simulink model "ExampleAnimationControl"  (Simulink 9.2)
settings: Solver=FixedStepDiscrete  StartTime=0.0  StopTime=inf  FixedStep=0.001  RelTol=1e-3  EnableMultiTasking=on
libraries: rFproPhysicsLib x6
settings Model: Creator=enewton  LastModifiedBy=AkinoriMinakawa
settings Model: SuppressorTable=|
  | <?xml version="1.0" encoding="UTF-8" standalone="yes" ?>
  | <!DOCTYPE boost_serialization>
  | <boost_serialization signature="serialization::archive" version="15">
  | <DiagnosticSuppressor class_id="0" tracking_level="0" version="6">
  | 	<Table class_id="1" tracking_level="0" version="0">
  | 		<count>4</count>
  | 		<bucket_count>8</bucket_count>
  | 		<item_version>0</item_version>
  | 		<item class_id="2" tracking_level="0" version="0">
  | 			<first class_id="3" tracking_level="0" version="6">
  | 				<Source class_id="4" tracking_level="0" version="0">
  | 					<count>1</count>
  | 					<item_version>0</item_version>
  | 					<item>ExampleAnimationControl/Insert Actor - Manual (state control)/Enable Send/Subsystem/Counter Free-Running2</item>
  | 				</Source>
  | 			</first>
  | 			<second class_id="5" tracking_level="0" version="6">
  | 				<SuppressedData class_id="6" tracking_level="0" version="0">
  | 					<count>2</count>
  | 					<bucket_count>8</bucket_count>
  | 					<item_version>0</item_version>
  | 					<item class_id="7" tracking_level="0" version="0">
  | 						<first class_id="8" tracking_level="0" version="6">
  | 							<ID>SimulinkFixedPoint:util:Overflowoccurred</ID>
  | 							<Cause>
  | 								<Source>
  | 									<count>0</count>
  | 									<item_version>0</item_version>
  | 								</Source>
  | 							</Cause>
  | 						</first>
  | 						<second class_id="9" tracking_level="0" version="6">
  | 							<Comment></Comment>
  | 							<User></User>
  | 							<LastModified class_id="10" tracking_level="0" version="0">
  | 								<ptime_date class_id="11" tracking_level="0" version="0">
  | 									<date>20160523</date>
  | 								</ptime_date>
  | 								<ptime_time_duration class_id="12" tracking_level="0" version="0">
  | 									<is_special>0</is_special>
  | 									<time_duration_hours>10</time_duration_hours>
  | 									<time_duration_minutes>57</time_duration_minutes>
  | 									<time_duration_seconds>55</time_duration_seconds>
  | 									<time_duration_fractional_seconds>0</time_duration_fractional_seconds>
  | 								</ptime_time_duration>
  | 							</LastModified>
  | 							<SuppressionType>1</SuppressionType>
  | 						</second>
  | 					</item>
  | 					<item>
  | 						<first>
  | 							<ID>Simulink:DataType:WarningOverFlowDetected</ID>
  | 							<Cause>
  | 								<Source>
  | 									<count>0</count>
  | 									<item_version>0</item_version>
  | 								</Source>
  | 							</Cause>
  | 						</first>
  | 						<second>
  | 							<Comment></Comment>
  | 							<User></User>
  | 							<LastModified>
  | 								<ptime_date>
  | 									<date>20160523</date>
  | 								</ptime_date>
  | 								<ptime_time_duration>
  | 									<is_special>0</is_special>
  | 									<time_duration_hours>10</time_duration_hours>
  | 									<time_duration_minutes>57</time_duration_minutes>
  | 									<time_duration_seconds>55</time_duration_seconds>
  | 									<time_duration_fractional_seconds>0</time_duration_fractional_seconds>
  | 								</ptime_time_duration>
  | 							</LastModified>
  | 							<SuppressionType>1</SuppressionType>
  | 						</second>
  | 					</item>
  | 				</SuppressedData>
  | 			</second>
  | 		</item>
  | 		<item>
  | 			<first>
  | 				<Source>
  | 					<count>1</count>
  | 					<item_version>0</item_version>
  | 					<item>ExampleAnimationControl/Insert Actor - Hybrid/Enable Send/Subsystem/Counter Free-Running2</item>
  | 				</Source>
  | 			</first>
  | 			<second>
  | 				<SuppressedData>
  | 					<count>2</count>
  | 					<bucket_count>8</bucket_count>
  | 					<item_version>0</item_version>
  | 					<item>
  | 						<first>
  | 							<ID>SimulinkFixedPoint:util:Overflowoccurred</ID>
  | 							<Cause>
  | 								<Source>
  | 									<count>0</count>
  | 									<item_version>0</item_version>
  | 								</Source>
  | 							</Cause>
  | 						</first>
  | 						<second>
  | 							<Comment></Comment>
  | 							<User></User>
  | 							<LastModified>
  | 								<ptime_date>
  | 									<date>20160523</date>
  | 								</ptime_date>
  | 								<ptime_time_duration>
  | 									<is_special>0</is_special>
  | 									<time_duration_hours>10</time_duration_hours>
  | 									<time_duration_minutes>57</time_duration_minutes>
  | 									<time_duration_seconds>55</time_duration_seconds>
  | 									<time_duration_fractional_seconds>0</time_duration_fractional_seconds>
  | 								</ptime_time_duration>
  | 							</LastModified>
  | 							<SuppressionType>1</SuppressionType>
  | 						</second>
  | 					</item>
  | 					<item>
  | 						<first>
  | 							<ID>Simulink:DataType:WarningOverFlowDetected</ID>
  | 							<Cause>
  | 								<Source>
  | 									<count>0</count>
  | 									<item_version>0</item_version>
  | 								</Source>
  | 							</Cause>
  | 						</first>
  | 						<second>
  | 							<Comment></Comment>
  | 							<User></User>
  | 							<LastModified>
  | 								<ptime_date>
  | 									<date>20160523</date>
  | 								</ptime_date>
  | 								<ptime_time_duration>
  | 									<is_special>0</is_special>
  | 									<time_duration_hours>10</time_duration_hours>
  | 									<time_duration_minutes>57</time_duration_minutes>
  | 									<time_duration_seconds>55</time_duration_seconds>
  | 									<time_duration_fractional_seconds>0</time_duration_fractional_seconds>
  | 								</ptime_time_duration>
  | 							</LastModified>
  | 							<SuppressionType>1</SuppressionType>
  | 						</second>
  | 					</item>
  | 				</SuppressedData>
  | 			</second>
  | 		</item>
  | 		<item>
  | 			<first>
  | 				<Source>
  | 					<count>1</count>
  | 					<item_version>0</item_version>
  | 					<item>ExampleAnimationControl/Physics Visualisation/Enable Pulse/Subsystem/Counter Free-Running2</item>
  | 				</Source>
  | 			</first>
  | 			<second>
  | 				<SuppressedData>
  | 					<count>2</count>
  | 					<bucket_count>8</bucket_count>
  | 					<item_version>0</item_version>
  | 					<item>
  | 						<first>
  | 							<ID>SimulinkFixedPoint:util:Overflowoccurred</ID>
  | 							<Cause>
  | 								<Source>
  | 									<count>0</count>
  | 									<item_version>0</item_version>
  | 								</Source>
  | 							</Cause>
  | 						</first>
  | 						<second>
  | 							<Comment></Comment>
  | 							<User></User>
  | 							<LastModified>
  | 								<ptime_date>
  | 									<date>20160523</date>
  | 								</ptime_date>
  | 								<ptime_time_duration>
  | 									<is_special>0</is_special>
  | 									<time_duration_hours>10</time_duration_hours>
  | 									<time_duration_minutes>57</time_duration_minutes>
  | 									<time_duration_seconds>55</time_duration_seconds>
  | 									<time_duration_fractional_seconds>0</time_duration_fractional_seconds>
  | 								</ptime_time_duration>
  | 							</LastModified>
  | 							<SuppressionType>1</SuppressionType>
  | 						</second>
  | 					</item>
  | 					<item>
  | 						<first>
  | 							<ID>Simulink:DataType:WarningOverFlowDetected</ID>
  | 							<Cause>
  | 								<Source>
  | 									<count>0</count>
  | 									<item_version>0</item_version>
  | 								</Source>
  | 							</Cause>
  | 						</first>
  | 						<second>
  | 							<Comment></Comment>
  | 							<User></User>
  | 							<LastModified>
  | 								<ptime_date>
  | 									<date>20160523</date>
  | 								</ptime_date>
  | 								<ptime_time_duration>
  | 									<is_special>0</is_special>
  | 									<time_duration_hours>10</time_duration_hours>
  | 									<time_duration_minutes>57</time_duration_minutes>
  | 									<time_duration_seconds>55</time_duration_seconds>
  | 									<time_duration_fractional_seconds>0</time_duration_fractional_seconds>
  | 								</ptime_time_duration>
  | 							</LastModified>
  | 							<SuppressionType>1</SuppressionType>
  | 						</second>
  | 					</item>
  | 				</SuppressedData>
  | 			</second>
  | 		</item>
  | 		<item>
  | 			<first>
  | 				<Source>
  | 					<count>1</count>
  | 					<item_version>0</item_version>
  | 					<item>ExampleAnimationControl/Insert Actor - Manual (state &amp; frame control)/Enable Send/Subsystem/Counter Free-Running2</item>
  | 				</Source>
  | 			</first>
  | 			<second>
  | 				<SuppressedData>
  | 					<count>2</count>
  | 					<bucket_count>8</bucket_count>
  | 					<item_version>0</item_version>
  | 					<item>
  | 						<first>
  | 							<ID>SimulinkFixedPoint:util:Overflowoccurred</ID>
  | 							<Cause>
  | 								<Source>
  | 									<count>0</count>
  | 									<item_version>0</item_version>
  | 								</Source>
  | 							</Cause>
  | 						</first>
  | 						<second>
  | 							<Comment></Comment>
  | 							<User></User>
  | 							<LastModified>
  | 								<ptime_date>
  | 									<date>20160523</date>
  | 								</ptime_date>
  | 								<ptime_time_duration>
  | 									<is_special>0</is_special>
  | 									<time_duration_hours>10</time_duration_hours>
  | 									<time_duration_minutes>57</time_duration_minutes>
  | 									<time_duration_seconds>55</time_duration_seconds>
  | 									<time_duration_fractional_seconds>0</time_duration_fractional_seconds>
  | 								</ptime_time_duration>
  | 							</LastModified>
  | 							<SuppressionType>1</SuppressionType>
  | 						</second>
  | 					</item>
  | 					<item>
  | 						<first>
  | 							<ID>Simulink:DataType:WarningOverFlowDetected</ID>
  | 							<Cause>
  | 								<Source>
  | 									<count>0</count>
  | 									<item_version>0</item_version>
  | 								</Source>
  | 							</Cause>
  | 						</first>
  | 						<second>
  | 							<Comment></Comment>
  | 							<User></User>
  | 							<LastModified>
  | 								<ptime_date>
  | 									<date>20160523</date>
  | 								</ptime_date>
  | 								<ptime_time_duration>
  | 									<is_special>0</is_special>
  | 									<time_duration_hours>10</time_duration_hours>
  | 									<time_duration_minutes>57</time_duration_minutes>
  | 									<time_duration_seconds>55</time_duration_seconds>
  | 									<time_duration_fractional_seconds>0</time_duration_fractional_seconds>
  | 								</ptime_time_duration>
  | 							</LastModified>
  | 							<SuppressionType>1</SuppressionType>
  | 						</second>
  | 					</item>
  | 				</SuppressedData>
  | 			</second>
  | 		</item>
  | 	</Table>
  | </DiagnosticSuppressor>
  | </boost_serialization>
settings OptimizationCC: ExpressionDepthLimit=2147483647  LifeSpan=auto
settings DebuggingCC: SolverPrmCheckMsg=warning
settings RTWCC: SystemTargetFile=rfpro.tlc  MakeCommand="make_rtw OPTS=\"-DRUN_PHYSICS\""  TemplateMakefile=rfpro.tmf  Description=rFpro Target (Run Physics)  TargetLang=C++
settings STFCustomTargetCC: ModelReferenceCompliant=off  CombineOutputUpdateFcns=on  MatFileLogging=on  GRTInterface=off  SystemTargetFile=rfpro.tlc
settings GRTTargetCC: ModelReferenceCompliant=off  ParMdlRefBuildCompliant=off  CompOptLevelCompliant=off  ConcurrentExecutionCompliant=off  GeneratePreprocessorConditionals=Use local settings  CombineOutputUpdateFcns=on  CPPClassGenCompliant=off  GRTInterface=off  UseToolchainInfoCompliant=off

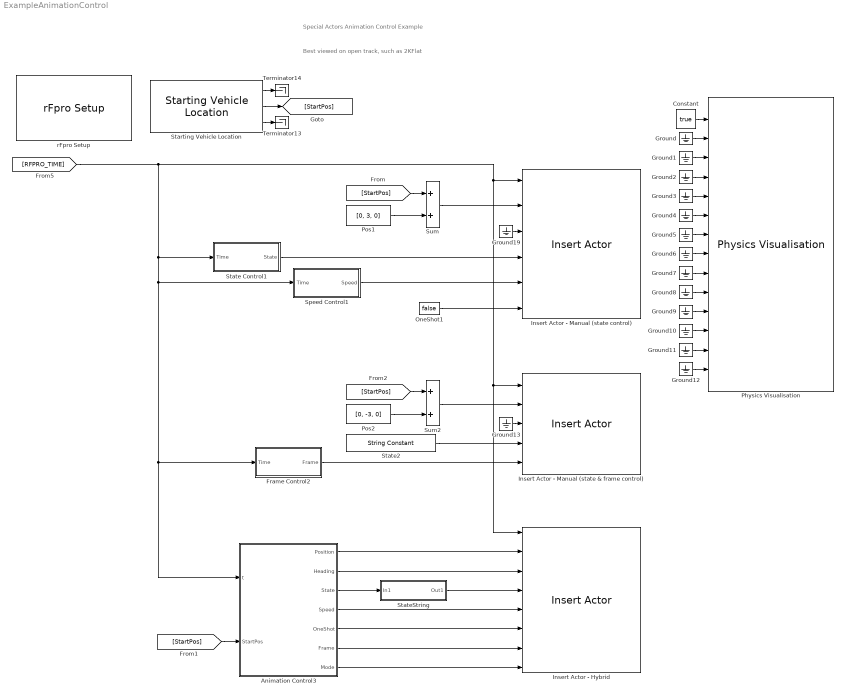
== system ExampleAnimationControl ==
  note: Special Actors Animation Control Example
  note: Best viewed on open track, such as 2KFlat
  Animation Control3 : MATLAB Function  TreatAsAtomicUnit=on
  Constant : Constant  Value=true
  Frame Control2 : Subsystem
  Ground{,1..13,19} (15 alike) : Ground
  Insert Actor - Hybrid : rFproPhysicsLib/Insert Actor  actorType='pedestrianMalcolmB'  instanceName=''  specialType=Pedestrian  doPreLoad=on  headingValid=on  heightValid=off  fixedHeight=0  relHeightFlag=on  orientationValid=off  animationControl=Hybrid  period=-1  offset=0  useReverseByteOrder=on  rFpro__platform=Remote Model - Default
  Insert Actor - Manual (state & frame control) : rFproPhysicsLib/Insert Actor  actorType='pedestrianMalcolmA'  instanceName=''  specialType=Pedestrian  doPreLoad=on  headingValid=off  heightValid=off  fixedHeight=0  relHeightFlag=on  orientationValid=off  animationControl=Manual (state & frame control)  period=-1  offset=0  useReverseByteOrder=on  rFpro__platform=Remote Model - Default
  Insert Actor - Manual (state control) : rFproPhysicsLib/Insert Actor  actorType='pedestrianMalcolmA'  instanceName=''  specialType=Pedestrian  doPreLoad=on  headingValid=off  heightValid=off  fixedHeight=0  relHeightFlag=on  orientationValid=off  animationControl=Manual (state control)  period=-1  offset=0  useReverseByteOrder=on  rFpro__platform=Remote Model - Default
  OneShot1 : Constant  Value=false
  Physics Visualisation : rFproPhysicsLib/Physics Visualisation  PAR_SKIP_INTERNAL_PHYSICS=off  PAR_ACCEL_VALID=off  PAR_ROT_ACCEL_VALID=off  PAR_GEAR_VALID=off  PAR_RPM_VALID=off  PAR_INPUTS_VALID=on  PAR_STEER_TORQUE_VALID=on  PAR_HEADLIGHTS_ON_VALID=off  PAR_WHEEL_POS_VALID=off  PAR_WHEEL_ORI_VALID=off  PAR_TYRE_PARAMS_VALID=off  PAR_WHEEL_ROTATION_VALID=off  PAR_WHEEL_BRAKE_TEMP_VALID=off  PAR_WHEEL_TREAD_TEMP_VALID=off  PAR_WHEEL_AIR_TEMP_VALID=off  period=-1  offset=0  useReverseByteOrder=on  rFpro__platform=Remote Model - Default
  Pos1 : Constant  Value=[0, 3, 0]
  Pos2 : Constant  Value=[0, -3, 0]
  Speed Control1 : Subsystem
  Starting Vehicle Location : rFproPhysicsLib/Starting Vehicle Location  cg_offset=[0, 0, 0]  numPackets=1  rFpro__platform=Remote Model - Default
  State Control1 : Subsystem
  State2 : StringConstant  String="\"fainting\""
  StateString : Subsystem
  Sum : Sum
  Sum2 : Sum
  Terminator13 : Terminator
  Terminator14 : Terminator
  rFpro Setup : rFproPhysicsLib/rFpro Setup  platform=Remote Model - Default  stopOnSessionEnd=on  usePseudoRealtime=on  syncToRF=on  useReverseByteOrder=off  useRfTime=on  minIterations=4  maxIterations=1000  ipReceiveAddress='127.0.0.1'  ipReceivePort=11054  receiveSampleTime=-1  ipTransmitAddress='127.0.0.1'  ipTransmitPort=11052  transmitSampleTime=-1  pluginType=RUN_PHYSICS  sysTarget=xpctarget.tlc  templateMakeFile=xpc_default_tmf  makeCommand=make_rtw  buildDesc=xPC target
  wires:
  Constant/1 -> Physics Visualisation/1
  Ground/1 -> Physics Visualisation/2
  Ground1/1 -> Physics Visualisation/3
  Ground2/1 -> Physics Visualisation/4
  Ground3/1 -> Physics Visualisation/5
  Ground4/1 -> Physics Visualisation/6
  Ground5/1 -> Physics Visualisation/7
  Ground6/1 -> Physics Visualisation/8
  Ground7/1 -> Physics Visualisation/9
  Ground8/1 -> Physics Visualisation/10
  Ground9/1 -> Physics Visualisation/11
  Ground10/1 -> Physics Visualisation/12
  Ground11/1 -> Physics Visualisation/13
  Ground12/1 -> Physics Visualisation/14
  Starting Vehicle Location/3 -> Terminator13/1
  Starting Vehicle Location/1 -> Terminator14/1
  Ground19/1 -> Insert Actor - Manual (state control)/3
  Sum/1 -> Insert Actor - Manual (state control)/2
  Pos1/1 -> Sum/2
  Starting Vehicle Location/2 -> [StartPos]
  [StartPos] -> Sum/1
  Speed Control1/1(Speed) -> Insert Actor - Manual (state control)/5
  OneShot1/1 -> Insert Actor - Manual (state control)/6
  State Control1/1(State) -> Insert Actor - Manual (state control)/4
  [RFPRO_TIME] -> State Control1/1(Time), Frame Control2/1(Time), Animation Control3/1(t), Speed Control1/1(Time), Insert Actor - Hybrid/1, Insert Actor - Manual (state & frame control)/1, Insert Actor - Manual (state control)/1
  Pos2/1 -> Sum2/2
  Sum2/1 -> Insert Actor - Manual (state & frame control)/2
  Ground13/1 -> Insert Actor - Manual (state & frame control)/3
  [StartPos] -> Sum2/1
  State2/1 -> Insert Actor - Manual (state & frame control)/4
  Animation Control3/2(Heading) -> Insert Actor - Hybrid/3
  Animation Control3/1(Position) -> Insert Actor - Hybrid/2
  Animation Control3/3(State) -> StateString/1(In1)
  Animation Control3/5(OneShot) -> Insert Actor - Hybrid/6
  Animation Control3/6(Frame) -> Insert Actor - Hybrid/7
  Animation Control3/7(Mode) -> Insert Actor - Hybrid/8
  StateString/1(Out1) -> Insert Actor - Hybrid/4
  Animation Control3/4(Speed) -> Insert Actor - Hybrid/5
  Frame Control2/1(Frame) -> Insert Actor - Manual (state & frame control)/5
  [StartPos] -> Animation Control3/2(StartPos)

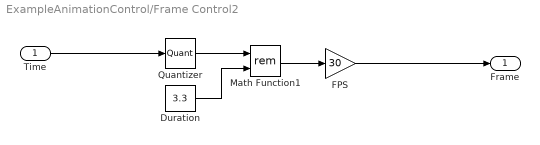
== system ExampleAnimationControl/Frame Control2 ==
  Time : Inport
  Duration : Constant  Value=3.3
  FPS : Gain  Gain=30
  Math Function1 : Math  Operator=rem  SaturateOnIntegerOverflow=on
  Quantizer : Quantizer
  Frame : Outport
  wires:
  Math Function1/1 -> FPS/1
  Quantizer/1 -> Math Function1/1
  Duration/1 -> Math Function1/2
  Time/1 -> Quantizer/1
  FPS/1 -> Frame/1

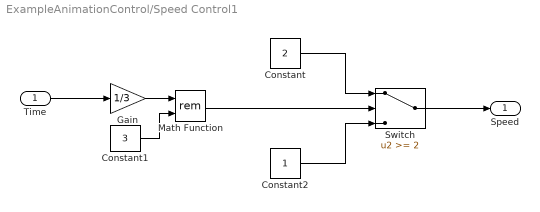
== system ExampleAnimationControl/Speed Control1 ==
  Time : Inport
  Constant : Constant  Value=2
  Constant1 : Constant  Value=3
  Constant2 : Constant
  Gain : Gain  Gain=1/3
  Math Function : Math  Operator=rem  SaturateOnIntegerOverflow=on
  Switch : Switch  Threshold=2
  Speed : Outport
  wires:
  Math Function/1 -> Switch/2
  Gain/1 -> Math Function/1
  Constant2/1 -> Switch/3
  Time/1 -> Gain/1
  Constant1/1 -> Math Function/2
  Constant/1 -> Switch/1
  Switch/1 -> Speed/1

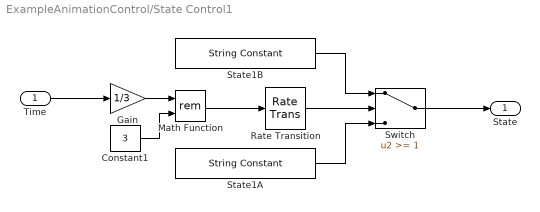
== system ExampleAnimationControl/State Control1 ==
  Time : Inport
  Constant1 : Constant  Value=3
  Gain : Gain  Gain=1/3
  Math Function : Math  Operator=rem  SaturateOnIntegerOverflow=on
  Rate Transition : RateTransition
  State1A : StringConstant  String="\"stretching\""
  State1B : StringConstant  String="\"walking\""
  Switch : Switch  Threshold=1
  State : Outport
  wires:
  Rate Transition/1 -> Switch/2
  Math Function/1 -> Rate Transition/1
  Gain/1 -> Math Function/1
  State1A/1 -> Switch/3
  Time/1 -> Gain/1
  Constant1/1 -> Math Function/2
  State1B/1 -> Switch/1
  Switch/1 -> State/1

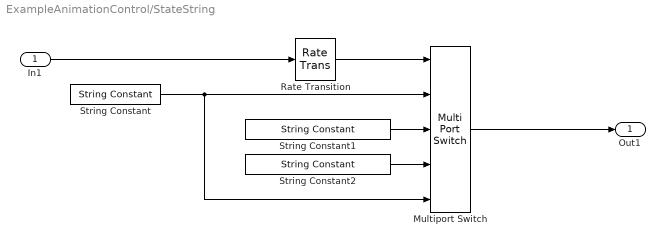
== system ExampleAnimationControl/StateString ==
  In1 : Inport
  Multiport Switch : MultiPortSwitch  DataPortOrder=Zero-based contiguous  DataPortForDefault=Additional data port  zeroidx=on
  Rate Transition : RateTransition
  String Constant : StringConstant  String="\"\""
  String Constant1 : StringConstant  String="\"tripping\""
  String Constant2 : StringConstant  String="\"fainting\""
  Out1 : Outport
  wires:
  In1/1 -> Rate Transition/1
  Multiport Switch/1 -> Out1/1
  String Constant/1 -> Multiport Switch/5, Multiport Switch/2
  String Constant1/1 -> Multiport Switch/3
  String Constant2/1 -> Multiport Switch/4
  Rate Transition/1 -> Multiport Switch/1

== matlab function Animation Control3 ==
  data: t input double; Position output double; Heading output double; State output double; Speed output double; OneShot output double; Frame output double; Mode output double; StartPos input double
function [Position, Heading, State, Speed, OneShot, Frame, Mode] = fcn(t, StartPos)

% StateString subsystem converts these numbers to strings
stateDefault = 0;
stateTrip = 1;
stateFaint = 2;

% Pedestrian movement definition
radius = 8;
vel = 1;

% Animation time
duration = 16;
loopCount = floor(t/duration);
loopTime = rem(t, duration);

% Set default output values to prevent variables from being left unset
State = stateDefault;
Speed = 1.0;
OneShot = true;
Frame = 0;

% Control the pedestrian with the hybrid animation mode
if loopTime < 4
    travelledDistance = 6*loopCount + vel*loopTime;
    
    Mode = 0;   % Automatic (speed-based)
elseif loopTime < 8
    travelledDistance = 6*loopCount + 4;
    
    Mode = 1;   % Manual (state control)
    State = stateTrip;
    Speed = 1.0;
    OneShot = true;
elseif loopTime < 12
    travelledDistance = 6*loopCount + 6;
    
    Mode = 0;   % Automatic (speed-based)
else
    travelledDistance = 6*loopCount + 6;
    
    Mode = 1;   % Manual (state control)
    State = stateFaint;
    Speed = 1.0;
    OneShot = true;
end

% Move the pedestrian in a circle
theta = travelledDistance / radius;
Position = radius * [cos(theta), sin(theta), 0] + StartPos;
Heading = theta + pi/2;
